simulink model "Basic_3DoF_Delta_2021a"  (R2021a)
settings: Solver=ode4  StartTime=0.0  StopTime=time(end)  FixedStep=0.001  RelTol=1e-6
model workspace: external: MATLAB File robot_6kg_v4_EXa5_DataFile.m (data not in the file)
values from neighbouring files (symbols this model uses):
  IAB = (Im + IA + IB)    [Basic_3DoF_Delta_Dynamic_Param.m]    (also in RL5_6kg_Dynamic_Param.m)
  IABe = (Im + IA + IBe)    [Basic_3DoF_Delta_Dynamic_Param.m]
  lB = l1*(rho1*m1 + me)    [Basic_3DoF_Delta_Dynamic_Param.m]    (also in RL5_6kg_Dynamic_Param.m)
  lBe = l1*(m1/2 + me)    [Basic_3DoF_Delta_Dynamic_Param.m]
  mD = m3 + 3*m2 + 3*me    [Basic_3DoF_Delta_Dynamic_Param.m]    (also in RL5_6kg_Dynamic_Param.m = m3 + 3*m2 + 3*me + mls_a4_spi + mls_a5_spi + mls_a5_worm)
  rho2 = Sro2    [Basic_3DoF_Delta_Dynamic_Param.m]    (also in RL5_6kg_Dynamic_Param.m)
undefined symbols (not defined in the file or in its folder): Inertias, X, Y, Z
libraries: sm_lib x119, nesl_utility x19, eeGeneralControl x3, simulink x3
(part 3 of 4)

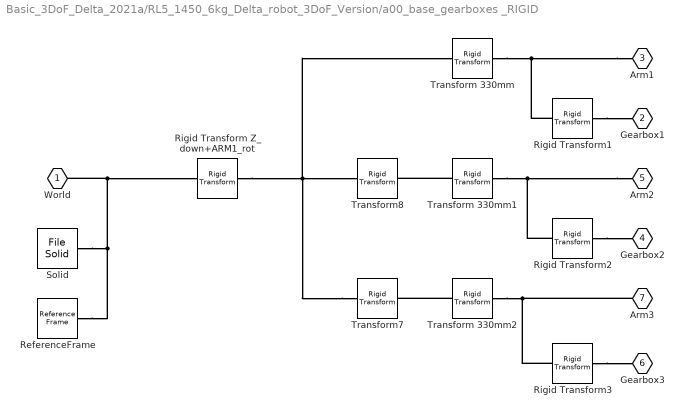
== system Basic_3DoF_Delta_2021a/RL5_1450_6kg_Delta_robot_3DoF_Version/a00_base_gearboxes _RIGID ==
  ReferenceFrame : sm_lib/Frames and Transforms/Reference Frame
  Rigid Transform1 : sm_lib/Frames and Transforms/Rigid Transform  TranslationMethod=Cartesian  TranslationStandardOffset=0  TranslationLengthUnit=mm  TranslationStandardAxis=+Z  TranslationCartesianOffset=[10 0 0]  TranslationROffset=0  TranslationROffsetUnits=m  TranslationZOffset=0  TranslationZOffsetUnits=m  TranslationThetaOffset=0  TranslationThetaOffsetUnits=deg  RotationMethod=None  RotationAngleUnits=deg  RotationStandardAxis=+Z  RotationAngle=0.0  RotationArbitraryAxis=[0 0 1]  FollAlignAxisA=+X  BaseAlignAxisA=+Y  FollAlignAxisB=+Y  BaseAlignAxisB=+Z  RotationSequenceAxes=FollowerAxes  RotationSequence=XYX  RotationSequenceAngles=[0 0 0]  RotationSequenceAnglesUnits=deg  RotationMatrix=[1 0 0; 0 1 0; 0 0 1]
  Rigid Transform2 : sm_lib/Frames and Transforms/Rigid Transform  TranslationMethod=Cartesian  TranslationStandardOffset=0  TranslationLengthUnit=mm  TranslationStandardAxis=+Z  TranslationCartesianOffset=[10 0 0]  TranslationROffset=0  TranslationROffsetUnits=m  TranslationZOffset=0  TranslationZOffsetUnits=m  TranslationThetaOffset=0  TranslationThetaOffsetUnits=deg  RotationMethod=None  RotationAngleUnits=deg  RotationStandardAxis=+Z  RotationAngle=0.0  RotationArbitraryAxis=[0 0 1]  FollAlignAxisA=+X  BaseAlignAxisA=+Y  FollAlignAxisB=+Y  BaseAlignAxisB=+Z  RotationSequenceAxes=FollowerAxes  RotationSequence=XYX  RotationSequenceAngles=[0 0 0]  RotationSequenceAnglesUnits=deg  RotationMatrix=[1 0 0; 0 1 0; 0 0 1]
  Rigid Transform3 : sm_lib/Frames and Transforms/Rigid Transform  TranslationMethod=Cartesian  TranslationStandardOffset=0  TranslationLengthUnit=mm  TranslationStandardAxis=+Z  TranslationCartesianOffset=[10 0 0]  TranslationROffset=0  TranslationROffsetUnits=m  TranslationZOffset=0  TranslationZOffsetUnits=m  TranslationThetaOffset=0  TranslationThetaOffsetUnits=deg  RotationMethod=None  RotationAngleUnits=deg  RotationStandardAxis=+Z  RotationAngle=0.0  RotationArbitraryAxis=[0 0 1]  FollAlignAxisA=+X  BaseAlignAxisA=+Y  FollAlignAxisB=+Y  BaseAlignAxisB=+Z  RotationSequenceAxes=FollowerAxes  RotationSequence=XYX  RotationSequenceAngles=[0 0 0]  RotationSequenceAnglesUnits=deg  RotationMatrix=[1 0 0; 0 1 0; 0 0 1]
  Rigid Transform Z_down+ARM1_rot : sm_lib/Frames and Transforms/Rigid Transform  TranslationMethod=None  TranslationStandardOffset=82.5  TranslationLengthUnit=mm  TranslationStandardAxis=-Z  TranslationCartesianOffset=[0 0 0]  TranslationROffset=0  TranslationROffsetUnits=m  TranslationZOffset=0  TranslationZOffsetUnits=m  TranslationThetaOffset=0  TranslationThetaOffsetUnits=deg  RotationMethod=AlignedAxes  RotationAngleUnits=deg  RotationStandardAxis=+X  RotationAngle=90  RotationArbitraryAxis=[0 0 1]  FollAlignAxisA=+Y  BaseAlignAxisA=+Z  FollAlignAxisB=+Z  BaseAlignAxisB=+Y  RotationSequenceAxes=BaseAxes  RotationSequence=XYX  RotationSequenceAngles=[-90 0 0]  RotationSequenceAnglesUnits=deg  RotationMatrix=[1 0 0; 0 1 0; 0 0 1]
  Solid : sm_lib/Body Elements/File Solid  ExtGeomFileName=a00_base_gearboxes.stp  UnitType=FromFile  ExtGeomFileUnits=m  StepReaderType=HEX  ExportConvexHullGeometry=off  InertiaType=CalculateFromGeometry  Mass=0  MassUnits=kg  CenterOfMass=0  CenterOfMassUnits=mm  MomentsOfInertia=0  MomentsOfInertiaUnits=kg*mm^2  ProductsOfInertia=0  ProductsOfInertiaUnits=kg*mm^2  BasedOnType=Density  Density=2345  DensityUnits=kg/m^3  DoExposeReferenceFrame=on  SerializedFrames=<Frames/>  GraphicType=FromGeometry  MarkerShape=Sphere  MarkerSize=10  GraphicVisPropType=SimpleVisualProperties  GraphicDiffuseColor=[0.6 0.6 0.6]  GraphicSpecularColor=[0.5 0.5 0.5 1.0]  GraphicAmbientColor=[0.15 0.15 0.15 1.0]  GraphicEmissiveColor=[0.0 0.0 0.0 1.0]  GraphicShininess=75  GraphicOpacity=1
  Transform 330mm : sm_lib/Frames and Transforms/Rigid Transform  TranslationMethod=StandardAxis  TranslationStandardOffset=330  TranslationLengthUnit=mm  TranslationStandardAxis=-X  TranslationCartesianOffset=0  TranslationROffset=0  TranslationROffsetUnits=m  TranslationZOffset=0  TranslationZOffsetUnits=m  TranslationThetaOffset=0  TranslationThetaOffsetUnits=deg  RotationMethod=AlignedAxes  RotationAngleUnits=rad  RotationStandardAxis=+Z  RotationAngle=0  RotationArbitraryAxis=0  FollAlignAxisA=+X  BaseAlignAxisA=+X  FollAlignAxisB=-Z  BaseAlignAxisB=+Z  RotationSequenceAxes=FollowerAxes  RotationSequence=XYX  RotationSequenceAngles=[-90 -60 180]  RotationSequenceAnglesUnits=deg  RotationMatrix=[1 0 0; 0 1 0; 0 0 1]
  Transform 330mm1 : sm_lib/Frames and Transforms/Rigid Transform  TranslationMethod=StandardAxis  TranslationStandardOffset=330  TranslationLengthUnit=mm  TranslationStandardAxis=-X  TranslationCartesianOffset=0  TranslationROffset=0  TranslationROffsetUnits=m  TranslationZOffset=0  TranslationZOffsetUnits=m  TranslationThetaOffset=0  TranslationThetaOffsetUnits=deg  RotationMethod=AlignedAxes  RotationAngleUnits=rad  RotationStandardAxis=+Z  RotationAngle=0  RotationArbitraryAxis=0  FollAlignAxisA=+X  BaseAlignAxisA=+X  FollAlignAxisB=-Z  BaseAlignAxisB=+Z  RotationSequenceAxes=FollowerAxes  RotationSequence=XYX  RotationSequenceAngles=[-90 -60 180]  RotationSequenceAnglesUnits=deg  RotationMatrix=[1 0 0; 0 1 0; 0 0 1]
  Transform 330mm2 : sm_lib/Frames and Transforms/Rigid Transform  TranslationMethod=StandardAxis  TranslationStandardOffset=330  TranslationLengthUnit=mm  TranslationStandardAxis=-X  TranslationCartesianOffset=0  TranslationROffset=0  TranslationROffsetUnits=m  TranslationZOffset=0  TranslationZOffsetUnits=m  TranslationThetaOffset=0  TranslationThetaOffsetUnits=deg  RotationMethod=AlignedAxes  RotationAngleUnits=rad  RotationStandardAxis=+Z  RotationAngle=0  RotationArbitraryAxis=0  FollAlignAxisA=+X  BaseAlignAxisA=+X  FollAlignAxisB=-Z  BaseAlignAxisB=+Z  RotationSequenceAxes=FollowerAxes  RotationSequence=XYX  RotationSequenceAngles=[-90 -60 180]  RotationSequenceAnglesUnits=deg  RotationMatrix=[1 0 0; 0 1 0; 0 0 1]
  Transform7 : sm_lib/Frames and Transforms/Rigid Transform  TranslationMethod=None  TranslationStandardOffset=0  TranslationLengthUnit=mm  TranslationStandardAxis=+Z  TranslationCartesianOffset=0  TranslationROffset=0  TranslationROffsetUnits=m  TranslationZOffset=0  TranslationZOffsetUnits=m  TranslationThetaOffset=0  TranslationThetaOffsetUnits=deg  RotationMethod=StandardAxis  RotationAngleUnits=deg  RotationStandardAxis=-Y  RotationAngle=120  RotationArbitraryAxis=0  FollAlignAxisA=+X  BaseAlignAxisA=+Y  FollAlignAxisB=+Y  BaseAlignAxisB=+Z  RotationSequenceAxes=FollowerAxes  RotationSequence=XZY  RotationSequenceAngles=[-90 180 0]  RotationSequenceAnglesUnits=deg  RotationMatrix=[1 0 0; 0 1 0; 0 0 1]
  Transform8 : sm_lib/Frames and Transforms/Rigid Transform  TranslationMethod=None  TranslationStandardOffset=0  TranslationLengthUnit=mm  TranslationStandardAxis=+Z  TranslationCartesianOffset=0  TranslationROffset=0  TranslationROffsetUnits=m  TranslationZOffset=0  TranslationZOffsetUnits=m  TranslationThetaOffset=0  TranslationThetaOffsetUnits=deg  RotationMethod=StandardAxis  RotationAngleUnits=deg  RotationStandardAxis=+Y  RotationAngle=120  RotationArbitraryAxis=0  FollAlignAxisA=+X  BaseAlignAxisA=+Y  FollAlignAxisB=+Y  BaseAlignAxisB=+Z  RotationSequenceAxes=FollowerAxes  RotationSequence=XYX  RotationSequenceAngles=[90 -60 0]  RotationSequenceAnglesUnits=deg  RotationMatrix=[1 0 0; 0 1 0; 0 0 1]
  World : PMIOPort  Side=Left
  Gearbox1 : PMIOPort  Port=2  Side=Right
  Arm1 : PMIOPort  Port=3  Side=Right
  Gearbox2 : PMIOPort  Port=4  Side=Right
  Arm2 : PMIOPort  Port=5  Side=Right
  Gearbox3 : PMIOPort  Port=6  Side=Right
  Arm3 : PMIOPort  Port=7  Side=Right
  connections:
  Solid/RConn1 -- World/RConn1 -- Rigid Transform Z_down+ARM1_rot/LConn1 -- ReferenceFrame/RConn1
  Arm1/RConn1 -- Rigid Transform1/LConn1 -- Transform 330mm/RConn1
  Rigid Transform3/LConn1 -- Transform 330mm2/RConn1 -- Arm3/RConn1
  Transform 330mm2/LConn1 -- Transform7/RConn1
  Arm2/RConn1 -- Transform 330mm1/RConn1 -- Rigid Transform2/LConn1
  Transform 330mm1/LConn1 -- Transform8/RConn1
  Transform7/LConn1 -- Transform8/LConn1 -- Transform 330mm/LConn1 -- Rigid Transform Z_down+ARM1_rot/RConn1
  Rigid Transform3/RConn1 -- Gearbox3/RConn1
  Rigid Transform2/RConn1 -- Gearbox2/RConn1
  Rigid Transform1/RConn1 -- Gearbox1/RConn1

== system Basic_3DoF_Delta_2021a/RL5_1450_6kg_Delta_robot_3DoF_Version/a00_gearbox_disk1_RIGID ==
  ReferenceFrame : sm_lib/Frames and Transforms/Reference Frame
  Solid(18) : sm_lib/Body Elements/File Solid  Description=Arm Reduced gearbox  ExtGeomFileName=a00_gearbox_disk.stp  UnitType=FromFile  ExtGeomFileUnits=m  StepReaderType=HEX  ExportConvexHullGeometry=off  InertiaType=Custom  Mass=0  MassUnits=kg  CenterOfMass=[0 0 0]  CenterOfMassUnits=m  MomentsOfInertia=[Inertias.Solid(18).MoI]  MomentsOfInertiaUnits=kg*m^2  ProductsOfInertia=[0 0 0]  ProductsOfInertiaUnits=kg*m^2  BasedOnType=Mass  Density=1000  DensityUnits=kg/m^3  DoExposeReferenceFrame=on  SerializedFrames=<Frames/>  GraphicType=FromGeometry  MarkerShape=Sphere  MarkerSize=10  GraphicVisPropType=SimpleVisualProperties  GraphicDiffuseColor=[0.65 0.5 0.5]  GraphicSpecularColor=[0.5 0.5 0.5 1.0]  GraphicAmbientColor=[0.15 0.15 0.15 1.0]  GraphicEmissiveColor=[0.0 0.0 0.0 1.0]  GraphicShininess=75  GraphicOpacity=1
      settings: AttributesFormatString=|
      | "%<Description>"
      | MoI: %<MomentsOfInertia> [%<MomentsOfInertiaUnits>]
  Transform : sm_lib/Frames and Transforms/Rigid Transform  TranslationMethod=StandardAxis  TranslationStandardOffset=190  TranslationLengthUnit=mm  TranslationStandardAxis=-Z  TranslationCartesianOffset=0  TranslationROffset=0  TranslationROffsetUnits=m  TranslationZOffset=0  TranslationZOffsetUnits=m  TranslationThetaOffset=0  TranslationThetaOffsetUnits=deg  RotationMethod=None  RotationAngleUnits=rev  RotationStandardAxis=+X  RotationAngle=0.5  RotationArbitraryAxis=0  FollAlignAxisA=+X  BaseAlignAxisA=+Y  FollAlignAxisB=+Y  BaseAlignAxisB=+Z  RotationSequenceAxes=FollowerAxes  RotationSequence=XYX  RotationSequenceAngles=[0 0 0]  RotationSequenceAnglesUnits=deg  RotationMatrix=[1 0 0; 0 1 0; 0 0 1]
  B.Frame : PMIOPort  Side=Left
  connections:
  Transform/RConn1 -- B.Frame/RConn1
  Solid(18)/RConn1 -- Transform/LConn1 -- ReferenceFrame/RConn1

== system Basic_3DoF_Delta_2021a/RL5_1450_6kg_Delta_robot_3DoF_Version/a00_gearbox_disk2_RIGID ==
  ReferenceFrame : sm_lib/Frames and Transforms/Reference Frame
  Solid(18) : sm_lib/Body Elements/File Solid  Description=Arm Reduced gearbox  ExtGeomFileName=a00_gearbox_disk.stp  UnitType=FromFile  ExtGeomFileUnits=m  StepReaderType=HEX  ExportConvexHullGeometry=off  InertiaType=Custom  Mass=0  MassUnits=kg  CenterOfMass=[0 0 0]  CenterOfMassUnits=m  MomentsOfInertia=[Inertias.Solid(18).MoI]  MomentsOfInertiaUnits=kg*m^2  ProductsOfInertia=[0 0 0]  ProductsOfInertiaUnits=kg*m^2  BasedOnType=Mass  Density=1000  DensityUnits=kg/m^3  DoExposeReferenceFrame=on  SerializedFrames=<Frames/>  GraphicType=FromGeometry  MarkerShape=Sphere  MarkerSize=10  GraphicVisPropType=SimpleVisualProperties  GraphicDiffuseColor=[0.65 0.5 0.5]  GraphicSpecularColor=[0.5 0.5 0.5 1.0]  GraphicAmbientColor=[0.15 0.15 0.15 1.0]  GraphicEmissiveColor=[0.0 0.0 0.0 1.0]  GraphicShininess=75  GraphicOpacity=1
      settings: AttributesFormatString=|
      | "%<Description>"
      | MoI: %<MomentsOfInertia> [%<MomentsOfInertiaUnits>]
  Transform : sm_lib/Frames and Transforms/Rigid Transform  TranslationMethod=StandardAxis  TranslationStandardOffset=190  TranslationLengthUnit=mm  TranslationStandardAxis=-Z  TranslationCartesianOffset=0  TranslationROffset=0  TranslationROffsetUnits=m  TranslationZOffset=0  TranslationZOffsetUnits=m  TranslationThetaOffset=0  TranslationThetaOffsetUnits=deg  RotationMethod=None  RotationAngleUnits=rev  RotationStandardAxis=+X  RotationAngle=0.5  RotationArbitraryAxis=0  FollAlignAxisA=+X  BaseAlignAxisA=+Y  FollAlignAxisB=+Y  BaseAlignAxisB=+Z  RotationSequenceAxes=FollowerAxes  RotationSequence=XYX  RotationSequenceAngles=[0 0 0]  RotationSequenceAnglesUnits=deg  RotationMatrix=[1 0 0; 0 1 0; 0 0 1]
  B.Frame : PMIOPort  Side=Left
  connections:
  Transform/RConn1 -- B.Frame/RConn1
  Solid(18)/RConn1 -- Transform/LConn1 -- ReferenceFrame/RConn1

== system Basic_3DoF_Delta_2021a/RL5_1450_6kg_Delta_robot_3DoF_Version/a00_gearbox_disk3_RIGID ==
  ReferenceFrame : sm_lib/Frames and Transforms/Reference Frame
  Solid(18) : sm_lib/Body Elements/File Solid  Description=Arm Reduced gearbox  ExtGeomFileName=a00_gearbox_disk.stp  UnitType=FromFile  ExtGeomFileUnits=m  StepReaderType=HEX  ExportConvexHullGeometry=off  InertiaType=Custom  Mass=0  MassUnits=kg  CenterOfMass=[0 0 0]  CenterOfMassUnits=m  MomentsOfInertia=[Inertias.Solid(18).MoI]  MomentsOfInertiaUnits=kg*m^2  ProductsOfInertia=[0 0 0]  ProductsOfInertiaUnits=kg*m^2  BasedOnType=Mass  Density=1000  DensityUnits=kg/m^3  DoExposeReferenceFrame=on  SerializedFrames=<Frames/>  GraphicType=FromGeometry  MarkerShape=Sphere  MarkerSize=10  GraphicVisPropType=SimpleVisualProperties  GraphicDiffuseColor=[0.65 0.5 0.5]  GraphicSpecularColor=[0.5 0.5 0.5 1.0]  GraphicAmbientColor=[0.15 0.15 0.15 1.0]  GraphicEmissiveColor=[0.0 0.0 0.0 1.0]  GraphicShininess=75  GraphicOpacity=1
      settings: AttributesFormatString=|
      | "%<Description>"
      | MoI: %<MomentsOfInertia> [%<MomentsOfInertiaUnits>]
  Transform : sm_lib/Frames and Transforms/Rigid Transform  TranslationMethod=StandardAxis  TranslationStandardOffset=190  TranslationLengthUnit=mm  TranslationStandardAxis=-Z  TranslationCartesianOffset=0  TranslationROffset=0  TranslationROffsetUnits=m  TranslationZOffset=0  TranslationZOffsetUnits=m  TranslationThetaOffset=0  TranslationThetaOffsetUnits=deg  RotationMethod=None  RotationAngleUnits=rev  RotationStandardAxis=+X  RotationAngle=0.5  RotationArbitraryAxis=0  FollAlignAxisA=+X  BaseAlignAxisA=+Y  FollAlignAxisB=+Y  BaseAlignAxisB=+Z  RotationSequenceAxes=FollowerAxes  RotationSequence=XYX  RotationSequenceAngles=[0 0 0]  RotationSequenceAnglesUnits=deg  RotationMatrix=[1 0 0; 0 1 0; 0 0 1]
  B.Frame : PMIOPort  Side=Left
  connections:
  Transform/RConn1 -- B.Frame/RConn1
  Solid(18)/RConn1 -- Transform/LConn1 -- ReferenceFrame/RConn1

== system Basic_3DoF_Delta_2021a/RL5_1450_6kg_Delta_robot_3DoF_Version/a01_upper_arm1 _RIGID ==
  ReferenceFrame : sm_lib/Frames and Transforms/Reference Frame
  Solid(2) : sm_lib/Body Elements/File Solid  Tag=Upper Arm  Description=Upper Arm  ExtGeomFileName=a01_upper_arm.stp  UnitType=FromFile  ExtGeomFileUnits=m  StepReaderType=HEX  ExportConvexHullGeometry=off  InertiaType=Custom  Mass=Inertias.Solid(2).mass  MassUnits=kg  CenterOfMass=Inertias.Solid(2).CoM  CenterOfMassUnits=m  MomentsOfInertia=Inertias.Solid(2).MoI  MomentsOfInertiaUnits=kg*m^2  ProductsOfInertia=Inertias.Solid(2).PoI  ProductsOfInertiaUnits=kg*m^2  BasedOnType=DensityFromFile  Density=1000  DensityUnits=kg/m^3  DoExposeReferenceFrame=on  SerializedFrames=<Frames/>  GraphicType=FromGeometry  MarkerShape=Sphere  MarkerSize=10  GraphicVisPropType=SimpleVisualProperties  GraphicDiffuseColor=[0.6 0.6 0.6]  GraphicSpecularColor=[0.5 0.5 0.5 1.0]  GraphicAmbientColor=[0.15 0.15 0.15 1.0]  GraphicEmissiveColor=[0.0 0.0 0.0 1.0]  GraphicShininess=75  GraphicOpacity=1
      settings: AttributesFormatString=|
      | "%<Description>"
      | Mass: %<Mass> [%<MassUnits>]
      | CoM: %<CenterOfMass> [%<CenterOfMassUnits>]
      | MoI: %<MomentsOfInertia> [%<MomentsOfInertiaUnits>]
      | PoI: %<ProductsOfInertia> [%<ProductsOfInertiaUnits>]
  Transform : sm_lib/Frames and Transforms/Rigid Transform  TranslationMethod=Cylindrical  TranslationStandardOffset=0  TranslationLengthUnit=mm  TranslationStandardAxis=+Z  TranslationCartesianOffset=0  TranslationROffset=420  TranslationROffsetUnits=mm  TranslationZOffset=0  TranslationZOffsetUnits=m  TranslationThetaOffset=5.327998  TranslationThetaOffsetUnits=deg  RotationMethod=AlignedAxes  RotationAngleUnits=rad  RotationStandardAxis=+Z  RotationAngle=0  RotationArbitraryAxis=0  FollAlignAxisA=+Z  BaseAlignAxisA=-Z  FollAlignAxisB=+X  BaseAlignAxisB=+X  RotationSequenceAxes=FollowerAxes  RotationSequence=XYX  RotationSequenceAngles=[0 0 0]  RotationSequenceAnglesUnits=deg  RotationMatrix=[1 0 0; 0 1 0; 0 0 1]
  B.frame : PMIOPort  Side=Left
  Forearm : PMIOPort  Port=2  Side=Right
  connections:
  Forearm/RConn1 -- ReferenceFrame/RConn1 -- Transform/LConn1 -- Solid(2)/RConn1
  Transform/RConn1 -- B.frame/RConn1

== system Basic_3DoF_Delta_2021a/RL5_1450_6kg_Delta_robot_3DoF_Version/a01_upper_arm2 _RIGID ==
  ReferenceFrame : sm_lib/Frames and Transforms/Reference Frame
  Solid(2) : sm_lib/Body Elements/File Solid  Tag=Upper Arm  Description=Upper Arm  ExtGeomFileName=a01_upper_arm.stp  UnitType=FromFile  ExtGeomFileUnits=m  StepReaderType=HEX  ExportConvexHullGeometry=off  InertiaType=Custom  Mass=Inertias.Solid(2).mass  MassUnits=kg  CenterOfMass=Inertias.Solid(2).CoM  CenterOfMassUnits=m  MomentsOfInertia=Inertias.Solid(2).MoI  MomentsOfInertiaUnits=kg*m^2  ProductsOfInertia=Inertias.Solid(2).PoI  ProductsOfInertiaUnits=kg*m^2  BasedOnType=DensityFromFile  Density=1000  DensityUnits=kg/m^3  DoExposeReferenceFrame=on  SerializedFrames=<Frames/>  GraphicType=FromGeometry  MarkerShape=Sphere  MarkerSize=10  GraphicVisPropType=SimpleVisualProperties  GraphicDiffuseColor=[0.6 0.6 0.6]  GraphicSpecularColor=[0.5 0.5 0.5 1.0]  GraphicAmbientColor=[0.15 0.15 0.15 1.0]  GraphicEmissiveColor=[0.0 0.0 0.0 1.0]  GraphicShininess=75  GraphicOpacity=1
      settings: AttributesFormatString=|
      | "%<Description>"
      | Mass: %<Mass> [%<MassUnits>]
      | CoM: %<CenterOfMass> [%<CenterOfMassUnits>]
      | MoI: %<MomentsOfInertia> [%<MomentsOfInertiaUnits>]
      | PoI: %<ProductsOfInertia> [%<ProductsOfInertiaUnits>]
  Transform : sm_lib/Frames and Transforms/Rigid Transform  TranslationMethod=Cylindrical  TranslationStandardOffset=0  TranslationLengthUnit=mm  TranslationStandardAxis=+Z  TranslationCartesianOffset=0  TranslationROffset=420  TranslationROffsetUnits=mm  TranslationZOffset=0  TranslationZOffsetUnits=m  TranslationThetaOffset=5.327998  TranslationThetaOffsetUnits=deg  RotationMethod=AlignedAxes  RotationAngleUnits=rad  RotationStandardAxis=+Z  RotationAngle=0  RotationArbitraryAxis=0  FollAlignAxisA=+Z  BaseAlignAxisA=-Z  FollAlignAxisB=+X  BaseAlignAxisB=+X  RotationSequenceAxes=FollowerAxes  RotationSequence=XYX  RotationSequenceAngles=[0 0 0]  RotationSequenceAnglesUnits=deg  RotationMatrix=[1 0 0; 0 1 0; 0 0 1]
  B.frame : PMIOPort  Side=Left
  Forearm : PMIOPort  Port=2  Side=Right
  connections:
  Forearm/RConn1 -- ReferenceFrame/RConn1 -- Transform/LConn1 -- Solid(2)/RConn1
  Transform/RConn1 -- B.frame/RConn1

== system Basic_3DoF_Delta_2021a/RL5_1450_6kg_Delta_robot_3DoF_Version/a01_upper_arm3 _RIGID ==
  ReferenceFrame : sm_lib/Frames and Transforms/Reference Frame
  Solid(2) : sm_lib/Body Elements/File Solid  Tag=Upper Arm  Description=Upper Arm  ExtGeomFileName=a01_upper_arm.stp  UnitType=FromFile  ExtGeomFileUnits=m  StepReaderType=HEX  ExportConvexHullGeometry=off  InertiaType=Custom  Mass=Inertias.Solid(2).mass  MassUnits=kg  CenterOfMass=Inertias.Solid(2).CoM  CenterOfMassUnits=m  MomentsOfInertia=Inertias.Solid(2).MoI  MomentsOfInertiaUnits=kg*m^2  ProductsOfInertia=Inertias.Solid(2).PoI  ProductsOfInertiaUnits=kg*m^2  BasedOnType=DensityFromFile  Density=1000  DensityUnits=kg/m^3  DoExposeReferenceFrame=on  SerializedFrames=<Frames/>  GraphicType=FromGeometry  MarkerShape=Sphere  MarkerSize=10  GraphicVisPropType=SimpleVisualProperties  GraphicDiffuseColor=[0.6 0.6 0.6]  GraphicSpecularColor=[0.5 0.5 0.5 1.0]  GraphicAmbientColor=[0.15 0.15 0.15 1.0]  GraphicEmissiveColor=[0.0 0.0 0.0 1.0]  GraphicShininess=75  GraphicOpacity=1
      settings: AttributesFormatString=|
      | "%<Description>"
      | Mass: %<Mass> [%<MassUnits>]
      | CoM: %<CenterOfMass> [%<CenterOfMassUnits>]
      | MoI: %<MomentsOfInertia> [%<MomentsOfInertiaUnits>]
      | PoI: %<ProductsOfInertia> [%<ProductsOfInertiaUnits>]
  Transform : sm_lib/Frames and Transforms/Rigid Transform  TranslationMethod=Cylindrical  TranslationStandardOffset=0  TranslationLengthUnit=mm  TranslationStandardAxis=+Z  TranslationCartesianOffset=0  TranslationROffset=420  TranslationROffsetUnits=mm  TranslationZOffset=0  TranslationZOffsetUnits=m  TranslationThetaOffset=5.327998  TranslationThetaOffsetUnits=deg  RotationMethod=AlignedAxes  RotationAngleUnits=rad  RotationStandardAxis=+Z  RotationAngle=0  RotationArbitraryAxis=0  FollAlignAxisA=+Z  BaseAlignAxisA=-Z  FollAlignAxisB=+X  BaseAlignAxisB=+X  RotationSequenceAxes=FollowerAxes  RotationSequence=XYX  RotationSequenceAngles=[0 0 0]  RotationSequenceAnglesUnits=deg  RotationMatrix=[1 0 0; 0 1 0; 0 0 1]
  B.frame : PMIOPort  Side=Left
  Forearm : PMIOPort  Port=2  Side=Right
  connections:
  Forearm/RConn1 -- ReferenceFrame/RConn1 -- Transform/LConn1 -- Solid(2)/RConn1
  Transform/RConn1 -- B.frame/RConn1

== system Basic_3DoF_Delta_2021a/RL5_1450_6kg_Delta_robot_3DoF_Version/a02_lower_arm1 _RIGID ==
  ReferenceFrame : sm_lib/Frames and Transforms/Reference Frame
  Solid(3) : sm_lib/Body Elements/File Solid  Description=Forearm  ExtGeomFileName=a02_lower_arm.stp  UnitType=FromFile  ExtGeomFileUnits=m  StepReaderType=HEX  ExportConvexHullGeometry=off  InertiaType=Custom  Mass=Inertias.Solid(3).mass  MassUnits=kg  CenterOfMass=Inertias.Solid(3).CoM  CenterOfMassUnits=m  MomentsOfInertia=Inertias.Solid(3).MoI  MomentsOfInertiaUnits=kg*m^2  ProductsOfInertia=Inertias.Solid(3).PoI  ProductsOfInertiaUnits=kg*m^2  BasedOnType=Mass  Density=1000  DensityUnits=kg/m^3  DoExposeReferenceFrame=on  SerializedFrames=<Frames/>  GraphicType=FromGeometry  MarkerShape=Sphere  MarkerSize=10  GraphicVisPropType=SimpleVisualProperties  GraphicDiffuseColor=[0.4 0.4 0.4]  GraphicSpecularColor=[0.5 0.5 0.5 1.0]  GraphicAmbientColor=[0.15 0.15 0.15 1.0]  GraphicEmissiveColor=[0.0 0.0 0.0 1.0]  GraphicShininess=75  GraphicOpacity=1
      settings: AttributesFormatString=|
      | "%<Description>"
      | Mass: %<Mass> [%<MassUnits>]
      | CoM: %<CenterOfMass> [%<CenterOfMassUnits>]
      | MoI: %<MomentsOfInertia> [%<MomentsOfInertiaUnits>]
      | PoI: %<ProductsOfInertia> [%<ProductsOfInertiaUnits>]
  Transform : sm_lib/Frames and Transforms/Rigid Transform  TranslationMethod=StandardAxis  TranslationStandardOffset=1055  TranslationLengthUnit=mm  TranslationStandardAxis=+X  TranslationCartesianOffset=0  TranslationROffset=0  TranslationROffsetUnits=m  TranslationZOffset=0  TranslationZOffsetUnits=m  TranslationThetaOffset=0  TranslationThetaOffsetUnits=deg  RotationMethod=StandardAxis  RotationAngleUnits=deg  RotationStandardAxis=-Z  RotationAngle=90  RotationArbitraryAxis=0  FollAlignAxisA=+X  BaseAlignAxisA=+Y  FollAlignAxisB=+Y  BaseAlignAxisB=+Z  RotationSequenceAxes=FollowerAxes  RotationSequence=XYX  RotationSequenceAngles=[0 0 0]  RotationSequenceAnglesUnits=deg  RotationMatrix=[1 0 0; 0 1 0; 0 0 1]
  Transform1 : sm_lib/Frames and Transforms/Rigid Transform  TranslationMethod=None  TranslationStandardOffset=0  TranslationLengthUnit=mm  TranslationStandardAxis=+Z  TranslationCartesianOffset=0  TranslationROffset=0  TranslationROffsetUnits=m  TranslationZOffset=0  TranslationZOffsetUnits=m  TranslationThetaOffset=0  TranslationThetaOffsetUnits=deg  RotationMethod=RotationSequence  RotationAngleUnits=rad  RotationStandardAxis=+Z  RotationAngle=0  RotationArbitraryAxis=0  FollAlignAxisA=+X  BaseAlignAxisA=+Y  FollAlignAxisB=+Y  BaseAlignAxisB=+Z  RotationSequenceAxes=FollowerAxes  RotationSequence=XZX  RotationSequenceAngles=[180 90 0]  RotationSequenceAnglesUnits=deg  RotationMatrix=[1 0 0; 0 1 0; 0 0 1]
  F1 : PMIOPort  Side=Left
  F : PMIOPort  Port=2  Side=Right
  connections:
  Transform1/RConn1 -- F1/RConn1
  Transform/RConn1 -- F/RConn1
  Transform1/LConn1 -- Solid(3)/RConn1 -- ReferenceFrame/RConn1 -- Transform/LConn1

== system Basic_3DoF_Delta_2021a/RL5_1450_6kg_Delta_robot_3DoF_Version/a02_lower_arm2 _RIGID ==
  ReferenceFrame : sm_lib/Frames and Transforms/Reference Frame
  Solid(3) : sm_lib/Body Elements/File Solid  Description=Forearm  ExtGeomFileName=a02_lower_arm.stp  UnitType=FromFile  ExtGeomFileUnits=m  StepReaderType=HEX  ExportConvexHullGeometry=off  InertiaType=Custom  Mass=Inertias.Solid(3).mass  MassUnits=kg  CenterOfMass=Inertias.Solid(3).CoM  CenterOfMassUnits=m  MomentsOfInertia=Inertias.Solid(3).MoI  MomentsOfInertiaUnits=kg*m^2  ProductsOfInertia=Inertias.Solid(3).PoI  ProductsOfInertiaUnits=kg*m^2  BasedOnType=Mass  Density=1000  DensityUnits=kg/m^3  DoExposeReferenceFrame=on  SerializedFrames=<Frames/>  GraphicType=FromGeometry  MarkerShape=Sphere  MarkerSize=10  GraphicVisPropType=SimpleVisualProperties  GraphicDiffuseColor=[0.4 0.4 0.4]  GraphicSpecularColor=[0.5 0.5 0.5 1.0]  GraphicAmbientColor=[0.15 0.15 0.15 1.0]  GraphicEmissiveColor=[0.0 0.0 0.0 1.0]  GraphicShininess=75  GraphicOpacity=1
      settings: AttributesFormatString=|
      | "%<Description>"
      | Mass: %<Mass> [%<MassUnits>]
      | CoM: %<CenterOfMass> [%<CenterOfMassUnits>]
      | MoI: %<MomentsOfInertia> [%<MomentsOfInertiaUnits>]
      | PoI: %<ProductsOfInertia> [%<ProductsOfInertiaUnits>]
  Transform : sm_lib/Frames and Transforms/Rigid Transform  TranslationMethod=StandardAxis  TranslationStandardOffset=1055  TranslationLengthUnit=mm  TranslationStandardAxis=+X  TranslationCartesianOffset=0  TranslationROffset=0  TranslationROffsetUnits=m  TranslationZOffset=0  TranslationZOffsetUnits=m  TranslationThetaOffset=0  TranslationThetaOffsetUnits=deg  RotationMethod=StandardAxis  RotationAngleUnits=deg  RotationStandardAxis=-Z  RotationAngle=90  RotationArbitraryAxis=0  FollAlignAxisA=+X  BaseAlignAxisA=+Y  FollAlignAxisB=+Y  BaseAlignAxisB=+Z  RotationSequenceAxes=FollowerAxes  RotationSequence=XYX  RotationSequenceAngles=[0 0 0]  RotationSequenceAnglesUnits=deg  RotationMatrix=[1 0 0; 0 1 0; 0 0 1]
  Transform1 : sm_lib/Frames and Transforms/Rigid Transform  TranslationMethod=None  TranslationStandardOffset=0  TranslationLengthUnit=mm  TranslationStandardAxis=+Z  TranslationCartesianOffset=0  TranslationROffset=0  TranslationROffsetUnits=m  TranslationZOffset=0  TranslationZOffsetUnits=m  TranslationThetaOffset=0  TranslationThetaOffsetUnits=deg  RotationMethod=RotationSequence  RotationAngleUnits=rad  RotationStandardAxis=+Z  RotationAngle=0  RotationArbitraryAxis=0  FollAlignAxisA=+X  BaseAlignAxisA=+Y  FollAlignAxisB=+Y  BaseAlignAxisB=+Z  RotationSequenceAxes=FollowerAxes  RotationSequence=XZX  RotationSequenceAngles=[180 90 0]  RotationSequenceAnglesUnits=deg  RotationMatrix=[1 0 0; 0 1 0; 0 0 1]
  F1 : PMIOPort  Side=Left
  F : PMIOPort  Port=2  Side=Right
  connections:
  Transform1/RConn1 -- F1/RConn1
  Transform/RConn1 -- F/RConn1
  Transform1/LConn1 -- ReferenceFrame/RConn1 -- Transform/LConn1 -- Solid(3)/RConn1

== system Basic_3DoF_Delta_2021a/RL5_1450_6kg_Delta_robot_3DoF_Version/a02_lower_arm3 _RIGID ==
  ReferenceFrame : sm_lib/Frames and Transforms/Reference Frame
  Solid(3) : sm_lib/Body Elements/File Solid  Description=Forearm  ExtGeomFileName=a02_lower_arm.stp  UnitType=FromFile  ExtGeomFileUnits=m  StepReaderType=HEX  ExportConvexHullGeometry=off  InertiaType=Custom  Mass=Inertias.Solid(3).mass  MassUnits=kg  CenterOfMass=Inertias.Solid(3).CoM  CenterOfMassUnits=m  MomentsOfInertia=Inertias.Solid(3).MoI  MomentsOfInertiaUnits=kg*m^2  ProductsOfInertia=Inertias.Solid(3).PoI  ProductsOfInertiaUnits=kg*m^2  BasedOnType=Mass  Density=1000  DensityUnits=kg/m^3  DoExposeReferenceFrame=on  SerializedFrames=<Frames/>  GraphicType=FromGeometry  MarkerShape=Sphere  MarkerSize=10  GraphicVisPropType=SimpleVisualProperties  GraphicDiffuseColor=[0.4 0.4 0.4]  GraphicSpecularColor=[0.5 0.5 0.5 1.0]  GraphicAmbientColor=[0.15 0.15 0.15 1.0]  GraphicEmissiveColor=[0.0 0.0 0.0 1.0]  GraphicShininess=75  GraphicOpacity=1
      settings: AttributesFormatString=|
      | "%<Description>"
      | Mass: %<Mass> [%<MassUnits>]
      | CoM: %<CenterOfMass> [%<CenterOfMassUnits>]
      | MoI: %<MomentsOfInertia> [%<MomentsOfInertiaUnits>]
      | PoI: %<ProductsOfInertia> [%<ProductsOfInertiaUnits>]
  Transform : sm_lib/Frames and Transforms/Rigid Transform  TranslationMethod=StandardAxis  TranslationStandardOffset=1055  TranslationLengthUnit=mm  TranslationStandardAxis=+X  TranslationCartesianOffset=0  TranslationROffset=0  TranslationROffsetUnits=m  TranslationZOffset=0  TranslationZOffsetUnits=m  TranslationThetaOffset=0  TranslationThetaOffsetUnits=deg  RotationMethod=StandardAxis  RotationAngleUnits=deg  RotationStandardAxis=-Z  RotationAngle=90  RotationArbitraryAxis=0  FollAlignAxisA=+X  BaseAlignAxisA=+Y  FollAlignAxisB=+Y  BaseAlignAxisB=+Z  RotationSequenceAxes=FollowerAxes  RotationSequence=XYX  RotationSequenceAngles=[0 0 0]  RotationSequenceAnglesUnits=deg  RotationMatrix=[1 0 0; 0 1 0; 0 0 1]
  Transform1 : sm_lib/Frames and Transforms/Rigid Transform  TranslationMethod=None  TranslationStandardOffset=0  TranslationLengthUnit=mm  TranslationStandardAxis=+Z  TranslationCartesianOffset=0  TranslationROffset=0  TranslationROffsetUnits=m  TranslationZOffset=0  TranslationZOffsetUnits=m  TranslationThetaOffset=0  TranslationThetaOffsetUnits=deg  RotationMethod=RotationSequence  RotationAngleUnits=rad  RotationStandardAxis=+Z  RotationAngle=0  RotationArbitraryAxis=0  FollAlignAxisA=+X  BaseAlignAxisA=+Y  FollAlignAxisB=+Y  BaseAlignAxisB=+Z  RotationSequenceAxes=FollowerAxes  RotationSequence=XZX  RotationSequenceAngles=[180 90 0]  RotationSequenceAnglesUnits=deg  RotationMatrix=[1 0 0; 0 1 0; 0 0 1]
  F1 : PMIOPort  Side=Left
  F : PMIOPort  Port=2  Side=Right
  connections:
  Transform1/RConn1 -- F1/RConn1
  Transform/RConn1 -- F/RConn1
  Transform1/LConn1 -- Solid(3)/RConn1 -- ReferenceFrame/RConn1 -- Transform/LConn1

== system Basic_3DoF_Delta_2021a/RL5_1450_6kg_Delta_robot_3DoF_Version/a02_lower_arm4 _RIGID ==
  ReferenceFrame : sm_lib/Frames and Transforms/Reference Frame
  Solid(3) : sm_lib/Body Elements/File Solid  Description=Forearm  ExtGeomFileName=a02_lower_arm.stp  UnitType=FromFile  ExtGeomFileUnits=m  StepReaderType=HEX  ExportConvexHullGeometry=off  InertiaType=Custom  Mass=Inertias.Solid(3).mass  MassUnits=kg  CenterOfMass=Inertias.Solid(3).CoM  CenterOfMassUnits=m  MomentsOfInertia=Inertias.Solid(3).MoI  MomentsOfInertiaUnits=kg*m^2  ProductsOfInertia=Inertias.Solid(3).PoI  ProductsOfInertiaUnits=kg*m^2  BasedOnType=Mass  Density=1000  DensityUnits=kg/m^3  DoExposeReferenceFrame=on  SerializedFrames=<Frames/>  GraphicType=FromGeometry  MarkerShape=Sphere  MarkerSize=10  GraphicVisPropType=SimpleVisualProperties  GraphicDiffuseColor=[0.4 0.4 0.4]  GraphicSpecularColor=[0.5 0.5 0.5 1.0]  GraphicAmbientColor=[0.15 0.15 0.15 1.0]  GraphicEmissiveColor=[0.0 0.0 0.0 1.0]  GraphicShininess=75  GraphicOpacity=1
      settings: AttributesFormatString=|
      | "%<Description>"
      | Mass: %<Mass> [%<MassUnits>]
      | CoM: %<CenterOfMass> [%<CenterOfMassUnits>]
      | MoI: %<MomentsOfInertia> [%<MomentsOfInertiaUnits>]
      | PoI: %<ProductsOfInertia> [%<ProductsOfInertiaUnits>]
  Transform : sm_lib/Frames and Transforms/Rigid Transform  TranslationMethod=StandardAxis  TranslationStandardOffset=1055  TranslationLengthUnit=mm  TranslationStandardAxis=+X  TranslationCartesianOffset=0  TranslationROffset=0  TranslationROffsetUnits=m  TranslationZOffset=0  TranslationZOffsetUnits=m  TranslationThetaOffset=0  TranslationThetaOffsetUnits=deg  RotationMethod=StandardAxis  RotationAngleUnits=deg  RotationStandardAxis=-Z  RotationAngle=90  RotationArbitraryAxis=0  FollAlignAxisA=+X  BaseAlignAxisA=+Y  FollAlignAxisB=+Y  BaseAlignAxisB=+Z  RotationSequenceAxes=FollowerAxes  RotationSequence=XYX  RotationSequenceAngles=[0 0 0]  RotationSequenceAnglesUnits=deg  RotationMatrix=[1 0 0; 0 1 0; 0 0 1]
  Transform1 : sm_lib/Frames and Transforms/Rigid Transform  TranslationMethod=None  TranslationStandardOffset=0  TranslationLengthUnit=mm  TranslationStandardAxis=+Z  TranslationCartesianOffset=0  TranslationROffset=0  TranslationROffsetUnits=m  TranslationZOffset=0  TranslationZOffsetUnits=m  TranslationThetaOffset=0  TranslationThetaOffsetUnits=deg  RotationMethod=RotationSequence  RotationAngleUnits=rad  RotationStandardAxis=+Z  RotationAngle=0  RotationArbitraryAxis=0  FollAlignAxisA=+X  BaseAlignAxisA=+Y  FollAlignAxisB=+Y  BaseAlignAxisB=+Z  RotationSequenceAxes=FollowerAxes  RotationSequence=XZX  RotationSequenceAngles=[180 90 0]  RotationSequenceAnglesUnits=deg  RotationMatrix=[1 0 0; 0 1 0; 0 0 1]
  F1 : PMIOPort  Side=Left
  F : PMIOPort  Port=2  Side=Right
  connections:
  Transform1/RConn1 -- F1/RConn1
  Transform/RConn1 -- F/RConn1
  ReferenceFrame/RConn1 -- Transform/LConn1 -- Transform1/LConn1 -- Solid(3)/RConn1

== system Basic_3DoF_Delta_2021a/RL5_1450_6kg_Delta_robot_3DoF_Version/a02_lower_arm5 _RIGID ==
  ReferenceFrame : sm_lib/Frames and Transforms/Reference Frame
  Solid(3) : sm_lib/Body Elements/File Solid  Description=Forearm  ExtGeomFileName=a02_lower_arm.stp  UnitType=FromFile  ExtGeomFileUnits=m  StepReaderType=HEX  ExportConvexHullGeometry=off  InertiaType=Custom  Mass=Inertias.Solid(3).mass  MassUnits=kg  CenterOfMass=Inertias.Solid(3).CoM  CenterOfMassUnits=m  MomentsOfInertia=Inertias.Solid(3).MoI  MomentsOfInertiaUnits=kg*m^2  ProductsOfInertia=Inertias.Solid(3).PoI  ProductsOfInertiaUnits=kg*m^2  BasedOnType=Mass  Density=1000  DensityUnits=kg/m^3  DoExposeReferenceFrame=on  SerializedFrames=<Frames/>  GraphicType=FromGeometry  MarkerShape=Sphere  MarkerSize=10  GraphicVisPropType=SimpleVisualProperties  GraphicDiffuseColor=[0.4 0.4 0.4]  GraphicSpecularColor=[0.5 0.5 0.5 1.0]  GraphicAmbientColor=[0.15 0.15 0.15 1.0]  GraphicEmissiveColor=[0.0 0.0 0.0 1.0]  GraphicShininess=75  GraphicOpacity=1
      settings: AttributesFormatString=|
      | "%<Description>"
      | Mass: %<Mass> [%<MassUnits>]
      | CoM: %<CenterOfMass> [%<CenterOfMassUnits>]
      | MoI: %<MomentsOfInertia> [%<MomentsOfInertiaUnits>]
      | PoI: %<ProductsOfInertia> [%<ProductsOfInertiaUnits>]
  Transform : sm_lib/Frames and Transforms/Rigid Transform  TranslationMethod=StandardAxis  TranslationStandardOffset=1055  TranslationLengthUnit=mm  TranslationStandardAxis=+X  TranslationCartesianOffset=0  TranslationROffset=0  TranslationROffsetUnits=m  TranslationZOffset=0  TranslationZOffsetUnits=m  TranslationThetaOffset=0  TranslationThetaOffsetUnits=deg  RotationMethod=StandardAxis  RotationAngleUnits=deg  RotationStandardAxis=-Z  RotationAngle=90  RotationArbitraryAxis=0  FollAlignAxisA=+X  BaseAlignAxisA=+Y  FollAlignAxisB=+Y  BaseAlignAxisB=+Z  RotationSequenceAxes=FollowerAxes  RotationSequence=XYX  RotationSequenceAngles=[0 0 0]  RotationSequenceAnglesUnits=deg  RotationMatrix=[1 0 0; 0 1 0; 0 0 1]
  Transform1 : sm_lib/Frames and Transforms/Rigid Transform  TranslationMethod=None  TranslationStandardOffset=0  TranslationLengthUnit=mm  TranslationStandardAxis=+Z  TranslationCartesianOffset=0  TranslationROffset=0  TranslationROffsetUnits=m  TranslationZOffset=0  TranslationZOffsetUnits=m  TranslationThetaOffset=0  TranslationThetaOffsetUnits=deg  RotationMethod=RotationSequence  RotationAngleUnits=rad  RotationStandardAxis=+Z  RotationAngle=0  RotationArbitraryAxis=0  FollAlignAxisA=+X  BaseAlignAxisA=+Y  FollAlignAxisB=+Y  BaseAlignAxisB=+Z  RotationSequenceAxes=FollowerAxes  RotationSequence=XZX  RotationSequenceAngles=[180 90 0]  RotationSequenceAnglesUnits=deg  RotationMatrix=[1 0 0; 0 1 0; 0 0 1]
  F1 : PMIOPort  Side=Left
  F : PMIOPort  Port=2  Side=Right
  connections:
  Transform1/RConn1 -- F1/RConn1
  Transform/RConn1 -- F/RConn1
  Transform1/LConn1 -- Solid(3)/RConn1 -- ReferenceFrame/RConn1 -- Transform/LConn1

== system Basic_3DoF_Delta_2021a/RL5_1450_6kg_Delta_robot_3DoF_Version/a02_lower_arm6 _RIGID ==
  ReferenceFrame : sm_lib/Frames and Transforms/Reference Frame
  Solid(3) : sm_lib/Body Elements/File Solid  Description=Forearm  ExtGeomFileName=a02_lower_arm.stp  UnitType=FromFile  ExtGeomFileUnits=m  StepReaderType=HEX  ExportConvexHullGeometry=off  InertiaType=Custom  Mass=Inertias.Solid(3).mass  MassUnits=kg  CenterOfMass=Inertias.Solid(3).CoM  CenterOfMassUnits=m  MomentsOfInertia=Inertias.Solid(3).MoI  MomentsOfInertiaUnits=kg*m^2  ProductsOfInertia=Inertias.Solid(3).PoI  ProductsOfInertiaUnits=kg*m^2  BasedOnType=Mass  Density=1000  DensityUnits=kg/m^3  DoExposeReferenceFrame=on  SerializedFrames=<Frames/>  GraphicType=FromGeometry  MarkerShape=Sphere  MarkerSize=10  GraphicVisPropType=SimpleVisualProperties  GraphicDiffuseColor=[0.4 0.4 0.4]  GraphicSpecularColor=[0.5 0.5 0.5 1.0]  GraphicAmbientColor=[0.15 0.15 0.15 1.0]  GraphicEmissiveColor=[0.0 0.0 0.0 1.0]  GraphicShininess=75  GraphicOpacity=1
      settings: AttributesFormatString=|
      | "%<Description>"
      | Mass: %<Mass> [%<MassUnits>]
      | CoM: %<CenterOfMass> [%<CenterOfMassUnits>]
      | MoI: %<MomentsOfInertia> [%<MomentsOfInertiaUnits>]
      | PoI: %<ProductsOfInertia> [%<ProductsOfInertiaUnits>]
  Transform : sm_lib/Frames and Transforms/Rigid Transform  TranslationMethod=StandardAxis  TranslationStandardOffset=1055  TranslationLengthUnit=mm  TranslationStandardAxis=+X  TranslationCartesianOffset=0  TranslationROffset=0  TranslationROffsetUnits=m  TranslationZOffset=0  TranslationZOffsetUnits=m  TranslationThetaOffset=0  TranslationThetaOffsetUnits=deg  RotationMethod=StandardAxis  RotationAngleUnits=deg  RotationStandardAxis=-Z  RotationAngle=90  RotationArbitraryAxis=0  FollAlignAxisA=+X  BaseAlignAxisA=+Y  FollAlignAxisB=+Y  BaseAlignAxisB=+Z  RotationSequenceAxes=FollowerAxes  RotationSequence=XYX  RotationSequenceAngles=[0 0 0]  RotationSequenceAnglesUnits=deg  RotationMatrix=[1 0 0; 0 1 0; 0 0 1]
  Transform1 : sm_lib/Frames and Transforms/Rigid Transform  TranslationMethod=None  TranslationStandardOffset=0  TranslationLengthUnit=mm  TranslationStandardAxis=+Z  TranslationCartesianOffset=0  TranslationROffset=0  TranslationROffsetUnits=m  TranslationZOffset=0  TranslationZOffsetUnits=m  TranslationThetaOffset=0  TranslationThetaOffsetUnits=deg  RotationMethod=RotationSequence  RotationAngleUnits=rad  RotationStandardAxis=+Z  RotationAngle=0  RotationArbitraryAxis=0  FollAlignAxisA=+X  BaseAlignAxisA=+Y  FollAlignAxisB=+Y  BaseAlignAxisB=+Z  RotationSequenceAxes=FollowerAxes  RotationSequence=XZX  RotationSequenceAngles=[180 90 0]  RotationSequenceAnglesUnits=deg  RotationMatrix=[1 0 0; 0 1 0; 0 0 1]
  F1 : PMIOPort  Side=Left
  F : PMIOPort  Port=2  Side=Right
  connections:
  Transform1/RConn1 -- F1/RConn1
  Transform/RConn1 -- F/RConn1
  ReferenceFrame/RConn1 -- Transform/LConn1 -- Transform1/LConn1 -- Solid(3)/RConn1

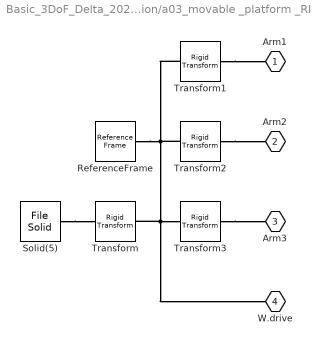
== system Basic_3DoF_Delta_2021a/RL5_1450_6kg_Delta_robot_3DoF_Version/a03_movable _platform _RIGID ==
  ReferenceFrame : sm_lib/Frames and Transforms/Reference Frame
  Solid(5) : sm_lib/Body Elements/File Solid  Description=Movable platform  ExtGeomFileName=a03_movable_platform.stp  UnitType=FromFile  ExtGeomFileUnits=m  StepReaderType=HEX  ExportConvexHullGeometry=off  InertiaType=Custom  Mass=Inertias.Solid(5).mass  MassUnits=kg  CenterOfMass=Inertias.Solid(5).CoM  CenterOfMassUnits=m  MomentsOfInertia=Inertias.Solid(5).MoI  MomentsOfInertiaUnits=kg*m^2  ProductsOfInertia=Inertias.Solid(5).PoI  ProductsOfInertiaUnits=kg*m^2  BasedOnType=Density  Density=3490  DensityUnits=kg/m^3  DoExposeReferenceFrame=on  SerializedFrames=<Frames/>  GraphicType=FromGeometry  MarkerShape=Sphere  MarkerSize=10  GraphicVisPropType=SimpleVisualProperties  GraphicDiffuseColor=[0.6 0.6 0.6]  GraphicSpecularColor=[0.5 0.5 0.5 1.0]  GraphicAmbientColor=[0.15 0.15 0.15 1.0]  GraphicEmissiveColor=[0.0 0.0 0.0 1.0]  GraphicShininess=75  GraphicOpacity=1
      settings: AttributesFormatString=|
      | "%<Description>"
      | Mass: %<Mass> [%<MassUnits>]
      | CoM: %<CenterOfMass> [%<CenterOfMassUnits>]
      | MoI: %<MomentsOfInertia> [%<MomentsOfInertiaUnits>]
      | PoI: %<ProductsOfInertia> [%<ProductsOfInertiaUnits>]
  Transform : sm_lib/Frames and Transforms/Rigid Transform  TranslationMethod=StandardAxis  TranslationStandardOffset=2.5  TranslationLengthUnit=mm  TranslationStandardAxis=-Z  TranslationCartesianOffset=0  TranslationROffset=0  TranslationROffsetUnits=m  TranslationZOffset=0  TranslationZOffsetUnits=m  TranslationThetaOffset=0  TranslationThetaOffsetUnits=deg  RotationMethod=RotationSequence  RotationAngleUnits=rad  RotationStandardAxis=+Z  RotationAngle=0  RotationArbitraryAxis=0  FollAlignAxisA=+X  BaseAlignAxisA=+Y  FollAlignAxisB=+Y  BaseAlignAxisB=+Z  RotationSequenceAxes=FollowerAxes  RotationSequence=ZXZ  RotationSequenceAngles=[-60 180 0]  RotationSequenceAnglesUnits=deg  RotationMatrix=[1 0 0; 0 1 0; 0 0 1]
  Transform1 : sm_lib/Frames and Transforms/Rigid Transform  TranslationMethod=Cylindrical  TranslationStandardOffset=47.5  TranslationLengthUnit=mm  TranslationStandardAxis=+Z  TranslationCartesianOffset=0  TranslationROffset=125  TranslationROffsetUnits=mm  TranslationZOffset=0  TranslationZOffsetUnits=m  TranslationThetaOffset=0  TranslationThetaOffsetUnits=deg  RotationMethod=StandardAxis  RotationAngleUnits=deg  RotationStandardAxis=+X  RotationAngle=90  RotationArbitraryAxis=0  FollAlignAxisA=+X  BaseAlignAxisA=+Y  FollAlignAxisB=+Y  BaseAlignAxisB=+Z  RotationSequenceAxes=FollowerAxes  RotationSequence=XYX  RotationSequenceAngles=[0 0 0]  RotationSequenceAnglesUnits=deg  RotationMatrix=[1 0 0; 0 1 0; 0 0 1]
  Transform2 : sm_lib/Frames and Transforms/Rigid Transform  TranslationMethod=Cylindrical  TranslationStandardOffset=47.5  TranslationLengthUnit=mm  TranslationStandardAxis=+Z  TranslationCartesianOffset=0  TranslationROffset=125  TranslationROffsetUnits=mm  TranslationZOffset=0  TranslationZOffsetUnits=m  TranslationThetaOffset=120  TranslationThetaOffsetUnits=deg  RotationMethod=RotationSequence  RotationAngleUnits=rad  RotationStandardAxis=+X  RotationAngle=90  RotationArbitraryAxis=0  FollAlignAxisA=+X  BaseAlignAxisA=+Y  FollAlignAxisB=+Y  BaseAlignAxisB=+Z  RotationSequenceAxes=FollowerAxes  RotationSequence=ZXZ  RotationSequenceAngles=[120 90 0]  RotationSequenceAnglesUnits=deg  RotationMatrix=[1 0 0; 0 1 0; 0 0 1]
  Transform3 : sm_lib/Frames and Transforms/Rigid Transform  TranslationMethod=Cylindrical  TranslationStandardOffset=47.5  TranslationLengthUnit=mm  TranslationStandardAxis=+Z  TranslationCartesianOffset=0  TranslationROffset=125  TranslationROffsetUnits=mm  TranslationZOffset=0  TranslationZOffsetUnits=m  TranslationThetaOffset=240  TranslationThetaOffsetUnits=deg  RotationMethod=RotationSequence  RotationAngleUnits=rad  RotationStandardAxis=+X  RotationAngle=90  RotationArbitraryAxis=0  FollAlignAxisA=+X  BaseAlignAxisA=+Y  FollAlignAxisB=+Y  BaseAlignAxisB=+Z  RotationSequenceAxes=FollowerAxes  RotationSequence=ZXZ  RotationSequenceAngles=[240 90 0]  RotationSequenceAnglesUnits=deg  RotationMatrix=[1 0 0; 0 1 0; 0 0 1]
  Arm1 : PMIOPort  Side=Left
  Arm2 : PMIOPort  Port=2  Side=Left
  Arm3 : PMIOPort  Port=3  Side=Left
  W.drive : PMIOPort  Port=4  Side=Right
  connections:
  Transform1/LConn1 -- Transform2/LConn1 -- Transform/RConn1 -- Transform3/LConn1 -- W.drive/RConn1 -- ReferenceFrame/RConn1
  Solid(5)/RConn1 -- Transform/LConn1
  Transform3/RConn1 -- Arm3/RConn1
  Transform2/RConn1 -- Arm2/RConn1
  Transform1/RConn1 -- Arm1/RConn1

== system Basic_3DoF_Delta_2021a/RL5_1450_6kg_Delta_robot_3DoF_Version/a16_pin1 _RIGID ==
  ReferenceFrame : sm_lib/Frames and Transforms/Reference Frame
  Solid(4) : sm_lib/Body Elements/File Solid  Description=Pin  ExtGeomFileName=a16_pin.stp  UnitType=FromFile  ExtGeomFileUnits=m  StepReaderType=HEX  ExportConvexHullGeometry=off  InertiaType=Custom  Mass=Inertias.Solid(4).mass  MassUnits=kg  CenterOfMass=Inertias.Solid(4).CoM  CenterOfMassUnits=m  MomentsOfInertia=Inertias.Solid(4).MoI  MomentsOfInertiaUnits=kg*m^2  ProductsOfInertia=Inertias.Solid(4).PoI  ProductsOfInertiaUnits=kg*m^2  BasedOnType=Density  Density=7850  DensityUnits=kg/m^3  DoExposeReferenceFrame=on  SerializedFrames=<Frames/>  GraphicType=FromGeometry  MarkerShape=Sphere  MarkerSize=10  GraphicVisPropType=SimpleVisualProperties  GraphicDiffuseColor=[0.8 0.8 0.8]  GraphicSpecularColor=[0.5 0.5 0.5 1.0]  GraphicAmbientColor=[0.15 0.15 0.15 1.0]  GraphicEmissiveColor=[0.0 0.0 0.0 1.0]  GraphicShininess=75  GraphicOpacity=1
      settings: AttributesFormatString=|
      | "%<Description>"
      | Mass: %<Mass> [%<MassUnits>]
      | CoM: %<CenterOfMass> [%<CenterOfMassUnits>]
      | MoI: %<MomentsOfInertia> [%<MomentsOfInertiaUnits>]
      | PoI: %<ProductsOfInertia> [%<ProductsOfInertiaUnits>]
  Transform : sm_lib/Frames and Transforms/Rigid Transform  TranslationMethod=StandardAxis  TranslationStandardOffset=67.5  TranslationLengthUnit=mm  TranslationStandardAxis=+X  TranslationCartesianOffset=0  TranslationROffset=0  TranslationROffsetUnits=m  TranslationZOffset=0  TranslationZOffsetUnits=m  TranslationThetaOffset=0  TranslationThetaOffsetUnits=deg  RotationMethod=StandardAxis  RotationAngleUnits=rad  RotationStandardAxis=+Z  RotationAngle=0  RotationArbitraryAxis=0  FollAlignAxisA=+X  BaseAlignAxisA=+Y  FollAlignAxisB=+Y  BaseAlignAxisB=+Z  RotationSequenceAxes=FollowerAxes  RotationSequence=XYX  RotationSequenceAngles=[0 0 0]  RotationSequenceAnglesUnits=deg  RotationMatrix=[1 0 0; 0 1 0; 0 0 1]
  Transform1 : sm_lib/Frames and Transforms/Rigid Transform  TranslationMethod=StandardAxis  TranslationStandardOffset=67.5  TranslationLengthUnit=mm  TranslationStandardAxis=-X  TranslationCartesianOffset=0  TranslationROffset=0  TranslationROffsetUnits=m  TranslationZOffset=0  TranslationZOffsetUnits=m  TranslationThetaOffset=0  TranslationThetaOffsetUnits=deg  RotationMethod=StandardAxis  RotationAngleUnits=deg  RotationStandardAxis=+Y  RotationAngle=180  RotationArbitraryAxis=0  FollAlignAxisA=+X  BaseAlignAxisA=+Y  FollAlignAxisB=+Y  BaseAlignAxisB=+Z  RotationSequenceAxes=FollowerAxes  RotationSequence=XYX  RotationSequenceAngles=[0 0 0]  RotationSequenceAnglesUnits=deg  RotationMatrix=[1 0 0; 0 1 0; 0 0 1]
  Transform2 : sm_lib/Frames and Transforms/Rigid Transform  TranslationMethod=None  TranslationStandardOffset=0  TranslationLengthUnit=mm  TranslationStandardAxis=+Z  TranslationCartesianOffset=0  TranslationROffset=0  TranslationROffsetUnits=m  TranslationZOffset=0  TranslationZOffsetUnits=m  TranslationThetaOffset=0  TranslationThetaOffsetUnits=deg  RotationMethod=StandardAxis  RotationAngleUnits=deg  RotationStandardAxis=+Y  RotationAngle=90  RotationArbitraryAxis=0  FollAlignAxisA=+X  BaseAlignAxisA=+Y  FollAlignAxisB=+Y  BaseAlignAxisB=+Z  RotationSequenceAxes=FollowerAxes  RotationSequence=XYX  RotationSequenceAngles=[0 0 0]  RotationSequenceAnglesUnits=deg  RotationMatrix=[1 0 0; 0 1 0; 0 0 1]
  Center : PMIOPort  Side=Left
  Link 1 : PMIOPort  Port=2  Side=Right
  Link 2 : PMIOPort  Port=3  Side=Right
  connections:
  Transform2/RConn1 -- Center/RConn1
  Transform1/RConn1 -- Link 1/RConn1
  Transform/RConn1 -- Link 2/RConn1
  Transform/LConn1 -- Transform1/LConn1 -- Transform2/LConn1 -- Solid(4)/RConn1 -- ReferenceFrame/RConn1
